simulink library "rtwdemo_pi_controller"  (Simulink 7.6)
settings: Solver=ode45  SolverMode=SingleTasking  StartTime=0.0  StopTime=10.0  RelTol=1e-3
undefined symbols (not defined in the file or in its folder): DiscIntNeverNeededParam, I_Gain, I_InErrMap, I_OutMap, P_Gain, P_InErrMap, P_OutMap
settings Model: Creator=The MathWorks Inc.  ExtModeAutoUpdateStatusClock=off

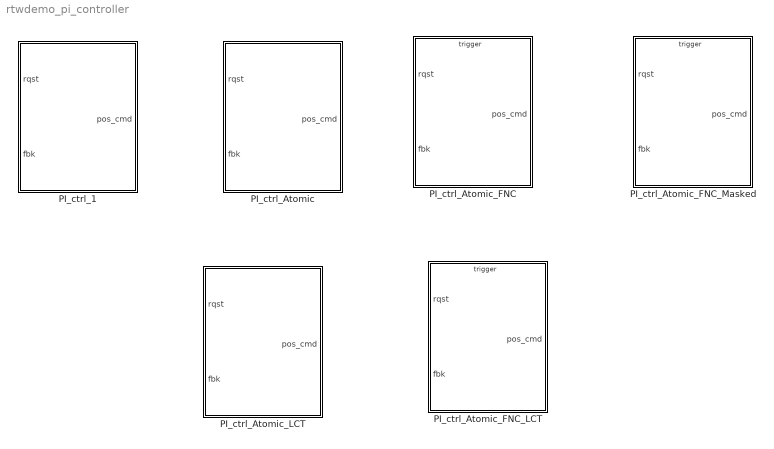
== system rtwdemo_pi_controller ==
  PI_ctrl_1 : Subsystem
      settings: RTWFileNameOpts=Use function name
  PI_ctrl_Atomic : Subsystem  TreatAsAtomicUnit=on  RTWFcnName=PI_Cntrl_Reusable
      settings: RTWFcnNameOpts=User specified  RTWFileNameOpts=Use function name
  PI_ctrl_Atomic_FNC : Subsystem  TreatAsAtomicUnit=on  RTWFcnName=PI_Cntrl_Reusable
      settings: RTWFcnNameOpts=User specified  RTWFileNameOpts=Use function name
  PI_ctrl_Atomic_FNC_LCT : Subsystem  TreatAsAtomicUnit=on  RTWFcnName=PI_Cntrl_Reusable
      settings: RTWFcnNameOpts=User specified  RTWFileNameOpts=Use function name
  PI_ctrl_Atomic_FNC_Masked : Subsystem  TreatAsAtomicUnit=on  RTWFcnName=PI_Cntrl_Reusable  mask{Masked_P_Gain=0, Masked_I_Gain=0}
      mask prompts: Masked_P_Gain "P_Gain"; Masked_I_Gain "I_Gain"
      settings: RTWFcnNameOpts=User specified  RTWFileNameOpts=Use function name
  PI_ctrl_Atomic_LCT : Subsystem  TreatAsAtomicUnit=on  RTWFcnName=PI_Cntrl_Reusable
      settings: RTWFcnNameOpts=User specified  RTWFileNameOpts=Use function name

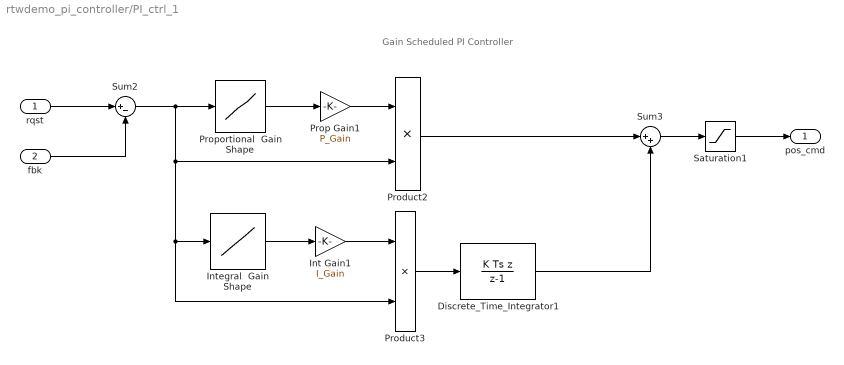
== system rtwdemo_pi_controller/PI_ctrl_1 ==
  note: Gain Scheduled PI Controller
  rqst : Inport
  fbk : Inport  Port=2
  Discrete_Time_Integrator1 : DiscreteIntegrator  IntegratorMethod=Integration: Backward Euler  InitialConditionMode=State only (most efficient)  SampleTime=-1  OutDataTypeStr=Inherit: Inherit via back propagation  UpperSaturationLimit=1  LowerSaturationLimit=-1  ICPrevOutput=DiscIntNeverNeededParam  ICPrevScaledInput=DiscIntNeverNeededParam
  Int Gain1 : Gain  Gain=I_Gain  OutDataTypeStr=Inherit: Same as input  ParamDataTypeStr=Inherit: Same as input
      settings: AttributesFormatString=%<Gain>
  Integral  Gain Shape : Lookup  InputValues=I_InErrMap  Table=I_OutMap
  Product2 : Product  RndMeth=Zero
  Product3 : Product  RndMeth=Zero
  Prop Gain1 : Gain  Gain=P_Gain  OutDataTypeStr=Inherit: Same as input  ParamDataTypeStr=Inherit: Same as input
      settings: AttributesFormatString=%<Gain>
  Proportional  Gain Shape : Lookup  InputValues=P_InErrMap  Table=P_OutMap
  Saturation1 : Saturate  UpperLimit=1  LowerLimit=-1
  Sum2 : Sum  Inputs=|+-  InputSameDT=on
  Sum3 : Sum  Inputs=|++  InputSameDT=on
  pos_cmd : Outport
  wires:
  Discrete_Time_Integrator1/1 -> Sum3/2
  Sum3/1 -> Saturation1/1
  Saturation1/1 -> pos_cmd/1
  rqst/1 -> Sum2/1
  fbk/1 -> Sum2/2
  Sum2/1 -> Product2/2, Product3/2, Integral  Gain Shape/1, Proportional  Gain Shape/1
  Integral  Gain Shape/1 -> Int Gain1/1
  Proportional  Gain Shape/1 -> Prop Gain1/1
  Int Gain1/1 -> Product3/1
  Product3/1 -> Discrete_Time_Integrator1/1
  Prop Gain1/1 -> Product2/1
  Product2/1 -> Sum3/1

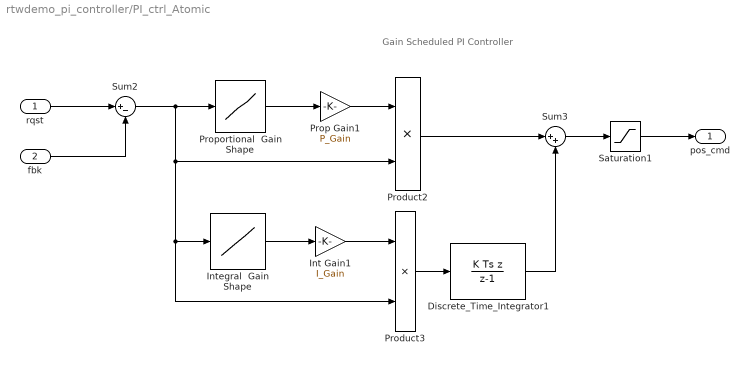
== system rtwdemo_pi_controller/PI_ctrl_Atomic ==
  note: Gain Scheduled PI Controller
  rqst : Inport
  fbk : Inport  Port=2
  Discrete_Time_Integrator1 : DiscreteIntegrator  IntegratorMethod=Integration: Backward Euler  InitialConditionMode=State only (most efficient)  SampleTime=-1  OutDataTypeStr=Inherit: Inherit via back propagation  UpperSaturationLimit=1  LowerSaturationLimit=-1  ICPrevOutput=DiscIntNeverNeededParam  ICPrevScaledInput=DiscIntNeverNeededParam
  Int Gain1 : Gain  Gain=I_Gain  OutDataTypeStr=Inherit: Same as input  ParamDataTypeStr=Inherit: Same as input
      settings: AttributesFormatString=%<Gain>
  Integral  Gain Shape : Lookup  InputValues=I_InErrMap  Table=I_OutMap
  Product2 : Product  RndMeth=Zero
  Product3 : Product  RndMeth=Zero
  Prop Gain1 : Gain  Gain=P_Gain  OutDataTypeStr=Inherit: Same as input  ParamDataTypeStr=Inherit: Same as input
      settings: AttributesFormatString=%<Gain>
  Proportional  Gain Shape : Lookup  InputValues=P_InErrMap  Table=P_OutMap
  Saturation1 : Saturate  UpperLimit=1  LowerLimit=-1
  Sum2 : Sum  Inputs=|+-  InputSameDT=on
  Sum3 : Sum  Inputs=|++  InputSameDT=on
  pos_cmd : Outport
  wires:
  Product2/1 -> Sum3/1
  Prop Gain1/1 -> Product2/1
  Product3/1 -> Discrete_Time_Integrator1/1
  Int Gain1/1 -> Product3/1
  Proportional  Gain Shape/1 -> Prop Gain1/1
  Integral  Gain Shape/1 -> Int Gain1/1
  Sum2/1 -> Proportional  Gain Shape/1, Integral  Gain Shape/1, Product3/2, Product2/2
  fbk/1 -> Sum2/2
  rqst/1 -> Sum2/1
  Saturation1/1 -> pos_cmd/1
  Sum3/1 -> Saturation1/1
  Discrete_Time_Integrator1/1 -> Sum3/2

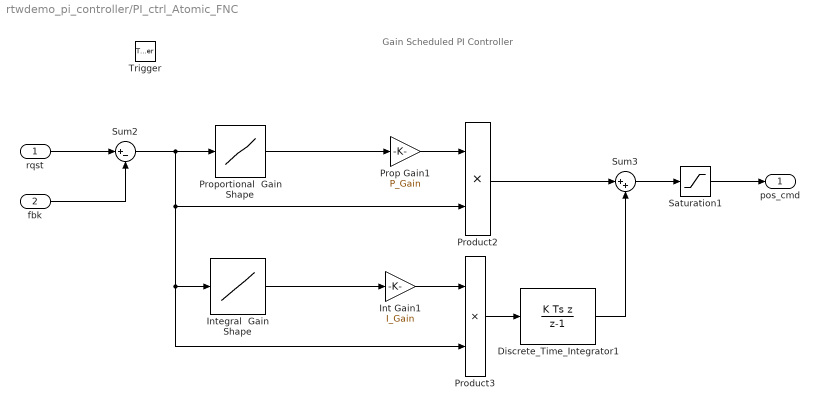
== system rtwdemo_pi_controller/PI_ctrl_Atomic_FNC ==
  note: Gain Scheduled PI Controller
  rqst : Inport
  fbk : Inport  Port=2
  Trigger : TriggerPort  TriggerType=function-call  SampleTimeType=periodic  SampleTime=.001
  Discrete_Time_Integrator1 : DiscreteIntegrator  IntegratorMethod=Integration: Backward Euler  InitialConditionMode=State only (most efficient)  SampleTime=-1  OutDataTypeStr=Inherit: Inherit via back propagation  UpperSaturationLimit=1  LowerSaturationLimit=-1  ICPrevOutput=DiscIntNeverNeededParam  ICPrevScaledInput=DiscIntNeverNeededParam
  Int Gain1 : Gain  Gain=I_Gain  OutDataTypeStr=Inherit: Same as input  ParamDataTypeStr=Inherit: Same as input
      settings: AttributesFormatString=%<Gain>
  Integral  Gain Shape : Lookup  InputValues=I_InErrMap  Table=I_OutMap
  Product2 : Product  RndMeth=Zero
  Product3 : Product  RndMeth=Zero
  Prop Gain1 : Gain  Gain=P_Gain  OutDataTypeStr=Inherit: Same as input  ParamDataTypeStr=Inherit: Same as input
      settings: AttributesFormatString=%<Gain>
  Proportional  Gain Shape : Lookup  InputValues=P_InErrMap  Table=P_OutMap
  Saturation1 : Saturate  UpperLimit=1  LowerLimit=-1
  Sum2 : Sum  Inputs=|+-  InputSameDT=on
  Sum3 : Sum  Inputs=|++  InputSameDT=on
  pos_cmd : Outport
  wires:
  Discrete_Time_Integrator1/1 -> Sum3/2
  Sum3/1 -> Saturation1/1
  Saturation1/1 -> pos_cmd/1
  rqst/1 -> Sum2/1
  fbk/1 -> Sum2/2
  Sum2/1 -> Product2/2, Product3/2, Integral  Gain Shape/1, Proportional  Gain Shape/1
  Integral  Gain Shape/1 -> Int Gain1/1
  Proportional  Gain Shape/1 -> Prop Gain1/1
  Int Gain1/1 -> Product3/1
  Product3/1 -> Discrete_Time_Integrator1/1
  Prop Gain1/1 -> Product2/1
  Product2/1 -> Sum3/1

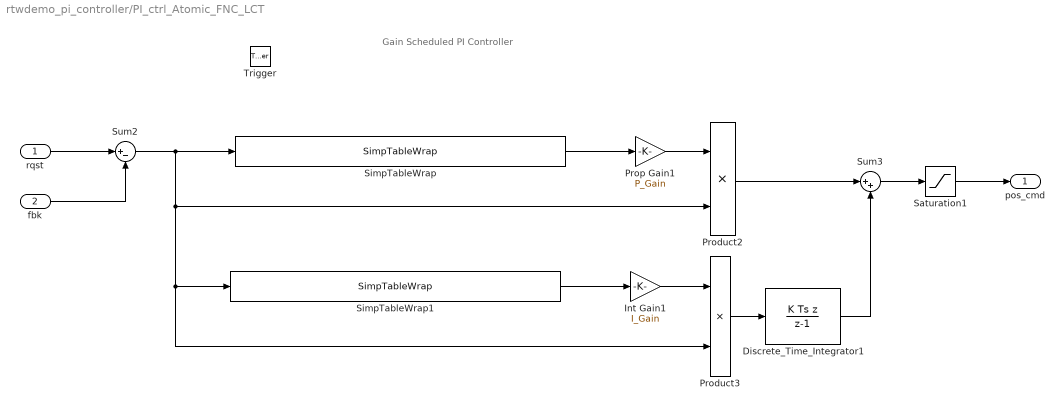
== system rtwdemo_pi_controller/PI_ctrl_Atomic_FNC_LCT ==
  note: Gain Scheduled PI Controller
  rqst : Inport
  fbk : Inport  Port=2
  Trigger : TriggerPort  TriggerType=function-call  SampleTimeType=periodic  SampleTime=.001
  Discrete_Time_Integrator1 : DiscreteIntegrator  IntegratorMethod=Integration: Backward Euler  InitialConditionMode=State only (most efficient)  SampleTime=-1  OutDataTypeStr=Inherit: Inherit via back propagation  UpperSaturationLimit=1  LowerSaturationLimit=-1  ICPrevOutput=DiscIntNeverNeededParam  ICPrevScaledInput=DiscIntNeverNeededParam
  Int Gain1 : Gain  Gain=I_Gain  OutDataTypeStr=Inherit: Same as input  ParamDataTypeStr=Inherit: Same as input
      settings: AttributesFormatString=%<Gain>
  Product2 : Product  RndMeth=Zero
  Product3 : Product  RndMeth=Zero
  Prop Gain1 : Gain  Gain=P_Gain  OutDataTypeStr=Inherit: Same as input  ParamDataTypeStr=Inherit: Same as input
      settings: AttributesFormatString=%<Gain>
  Saturation1 : Saturate  UpperLimit=1  LowerLimit=-1
  SimpTableWrap : S-Function  FunctionName=SimpTableWrap  Parameters=SParameter1, SParameter2, SParameter3  EnableBusSupport=off  mask(Legacy Function){SFunctionSpec=double y1 = SimpleTable(double u1, double p1[], double p2[], int16 p3), SParameter1=P_InErrMap, SParameter2=P_OutMap, SParameter3=int16(length(P_OutMap)), ShowSpec=on}
      mask prompts: SParameter1 "P1:"; SParameter2 "P2:"; SParameter3 "P3:"; ShowSpec "Display function specification"
      mask help:
      | This block allows the user to call the following C function(s) in Simulink:
      |
      | StartFcn: none
      |
      | OutputFcn: double y1 = SimpleTable(double u1, double p1[], double p2[], int16 p3)
      |
      | TerminateFcn: none
      mask CallbackString:
      | ||||if strcmp(get_param(gcbh, 'ShowSpec'), 'on')
      |   set_param(gcbh, 'MaskDisplay', sprintf('fprintf(''%s'');', get_param(gcbh, 'SFunctionSpec')));
      | else
      |   set_param(gcbh, 'MaskDisplay', sprintf('fprintf(''%s'');', get_param(gcbh, 'FunctionName')));
      | end
      mask Display: fprintf('double y1 = SimpleTable(double u1, double p1[], double p2[], int16 p3)');
  SimpTableWrap1 : S-Function  FunctionName=SimpTableWrap  Parameters=SParameter1, SParameter2, SParameter3  EnableBusSupport=off  mask(Legacy Function){SFunctionSpec=double y1 = SimpleTable(double u1, double p1[], double p2[], int16 p3), SParameter1=I_InErrMap, SParameter2=I_OutMap, SParameter3=int16(length(I_OutMap)), ShowSpec=on}
      mask prompts: SParameter1 "P1:"; SParameter2 "P2:"; SParameter3 "P3:"; ShowSpec "Display function specification"
      mask help:
      | This block allows the user to call the following C function(s) in Simulink:
      |
      | StartFcn: none
      |
      | OutputFcn: double y1 = SimpleTable(double u1, double p1[], double p2[], int16 p3)
      |
      | TerminateFcn: none
      mask CallbackString:
      | ||||if strcmp(get_param(gcbh, 'ShowSpec'), 'on')
      |   set_param(gcbh, 'MaskDisplay', sprintf('fprintf(''%s'');', get_param(gcbh, 'SFunctionSpec')));
      | else
      |   set_param(gcbh, 'MaskDisplay', sprintf('fprintf(''%s'');', get_param(gcbh, 'FunctionName')));
      | end
      mask Display: fprintf('double y1 = SimpleTable(double u1, double p1[], double p2[], int16 p3)');
  Sum2 : Sum  Inputs=|+-  InputSameDT=on
  Sum3 : Sum  Inputs=|++  InputSameDT=on
  pos_cmd : Outport
  wires:
  Product2/1 -> Sum3/1
  Prop Gain1/1 -> Product2/1
  Product3/1 -> Discrete_Time_Integrator1/1
  Int Gain1/1 -> Product3/1
  SimpTableWrap/1 -> Prop Gain1/1
  Sum2/1 -> Product2/2, Product3/2, SimpTableWrap1/1, SimpTableWrap/1
  fbk/1 -> Sum2/2
  rqst/1 -> Sum2/1
  Saturation1/1 -> pos_cmd/1
  Sum3/1 -> Saturation1/1
  Discrete_Time_Integrator1/1 -> Sum3/2
  SimpTableWrap1/1 -> Int Gain1/1

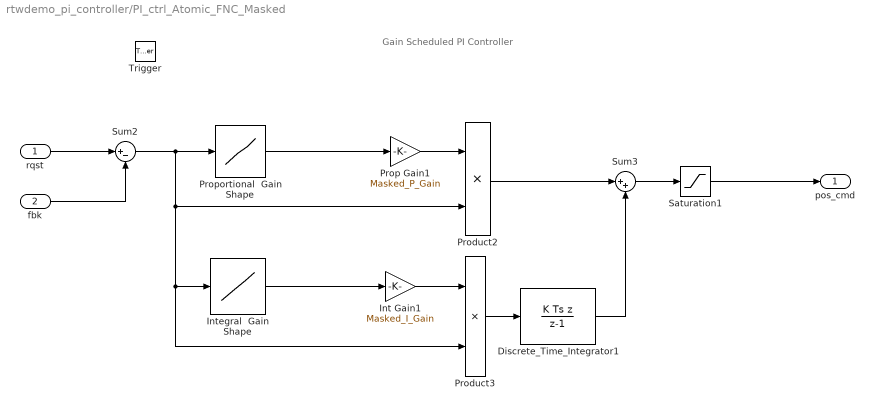
== system rtwdemo_pi_controller/PI_ctrl_Atomic_FNC_Masked ==
  note: Gain Scheduled PI Controller
  rqst : Inport
  fbk : Inport  Port=2
  Trigger : TriggerPort  TriggerType=function-call  SampleTimeType=periodic  SampleTime=.001
  Discrete_Time_Integrator1 : DiscreteIntegrator  IntegratorMethod=Integration: Backward Euler  InitialConditionMode=State only (most efficient)  SampleTime=-1  OutDataTypeStr=Inherit: Inherit via back propagation  UpperSaturationLimit=1  LowerSaturationLimit=-1  ICPrevOutput=DiscIntNeverNeededParam  ICPrevScaledInput=DiscIntNeverNeededParam
  Int Gain1 : Gain  Gain=Masked_I_Gain  OutDataTypeStr=Inherit: Same as input  ParamDataTypeStr=Inherit: Same as input
      settings: AttributesFormatString=%<Gain>
  Integral  Gain Shape : Lookup  InputValues=I_InErrMap  Table=I_OutMap
  Product2 : Product  RndMeth=Zero
  Product3 : Product  RndMeth=Zero
  Prop Gain1 : Gain  Gain=Masked_P_Gain  OutDataTypeStr=Inherit: Same as input  ParamDataTypeStr=Inherit: Same as input
      settings: AttributesFormatString=%<Gain>
  Proportional  Gain Shape : Lookup  InputValues=P_InErrMap  Table=P_OutMap
  Saturation1 : Saturate  UpperLimit=1  LowerLimit=-1
  Sum2 : Sum  Inputs=|+-  InputSameDT=on
  Sum3 : Sum  Inputs=|++  InputSameDT=on
  pos_cmd : Outport
  wires:
  Product2/1 -> Sum3/1
  Prop Gain1/1 -> Product2/1
  Product3/1 -> Discrete_Time_Integrator1/1
  Int Gain1/1 -> Product3/1
  Proportional  Gain Shape/1 -> Prop Gain1/1
  Integral  Gain Shape/1 -> Int Gain1/1
  Sum2/1 -> Proportional  Gain Shape/1, Integral  Gain Shape/1, Product3/2, Product2/2
  fbk/1 -> Sum2/2
  rqst/1 -> Sum2/1
  Saturation1/1 -> pos_cmd/1
  Sum3/1 -> Saturation1/1
  Discrete_Time_Integrator1/1 -> Sum3/2

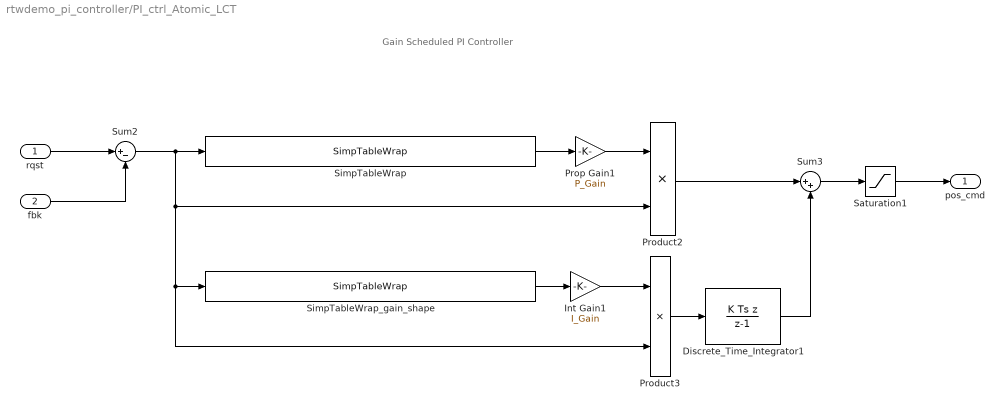
== system rtwdemo_pi_controller/PI_ctrl_Atomic_LCT ==
  note: Gain Scheduled PI Controller
  rqst : Inport
  fbk : Inport  Port=2
  Discrete_Time_Integrator1 : DiscreteIntegrator  IntegratorMethod=Integration: Backward Euler  InitialConditionMode=State only (most efficient)  SampleTime=-1  OutDataTypeStr=Inherit: Inherit via back propagation  UpperSaturationLimit=1  LowerSaturationLimit=-1  ICPrevOutput=DiscIntNeverNeededParam  ICPrevScaledInput=DiscIntNeverNeededParam
  Int Gain1 : Gain  Gain=I_Gain  OutDataTypeStr=Inherit: Same as input  ParamDataTypeStr=Inherit: Same as input
      settings: AttributesFormatString=%<Gain>
  Product2 : Product  RndMeth=Zero
  Product3 : Product  RndMeth=Zero
  Prop Gain1 : Gain  Gain=P_Gain  OutDataTypeStr=Inherit: Same as input  ParamDataTypeStr=Inherit: Same as input
      settings: AttributesFormatString=%<Gain>
  Saturation1 : Saturate  UpperLimit=1  LowerLimit=-1
  SimpTableWrap : S-Function  FunctionName=SimpTableWrap  Parameters=SParameter1, SParameter2, SParameter3  EnableBusSupport=off  mask(Legacy Function){SFunctionSpec=double y1 = SimpleTable(double u1, double p1[], double p2[], int16 p3), SParameter1=P_InErrMap, SParameter2=P_OutMap, SParameter3=int16(length(P_OutMap)), ShowSpec=on}
      mask prompts: SParameter1 "P1:"; SParameter2 "P2:"; SParameter3 "P3:"; ShowSpec "Display function specification"
      mask help:
      | This block allows the user to call the following C function(s) in Simulink:
      |
      | StartFcn: none
      |
      | OutputFcn: double y1 = SimpleTable(double u1, double p1[], double p2[], int16 p3)
      |
      | TerminateFcn: none
      mask CallbackString:
      | ||||if strcmp(get_param(gcbh, 'ShowSpec'), 'on')
      |   set_param(gcbh, 'MaskDisplay', sprintf('fprintf(''%s'');', get_param(gcbh, 'SFunctionSpec')));
      | else
      |   set_param(gcbh, 'MaskDisplay', sprintf('fprintf(''%s'');', get_param(gcbh, 'FunctionName')));
      | end
      mask Display: fprintf('double y1 = SimpleTable(double u1, double p1[], double p2[], int16 p3)');
  SimpTableWrap_gain_shape : S-Function  FunctionName=SimpTableWrap  Parameters=SParameter1, SParameter2, SParameter3  EnableBusSupport=off  mask(Legacy Function){SFunctionSpec=double y1 = SimpleTable(double u1, double p1[], double p2[], int16 p3), SParameter1=I_InErrMap, SParameter2=I_OutMap, SParameter3=int16(length(I_OutMap)), ShowSpec=on}
      mask prompts: SParameter1 "P1:"; SParameter2 "P2:"; SParameter3 "P3:"; ShowSpec "Display function specification"
      mask help:
      | This block allows the user to call the following C function(s) in Simulink:
      |
      | StartFcn: none
      |
      | OutputFcn: double y1 = SimpleTable(double u1, double p1[], double p2[], int16 p3)
      |
      | TerminateFcn: none
      mask CallbackString:
      | ||||if strcmp(get_param(gcbh, 'ShowSpec'), 'on')
      |   set_param(gcbh, 'MaskDisplay', sprintf('fprintf(''%s'');', get_param(gcbh, 'SFunctionSpec')));
      | else
      |   set_param(gcbh, 'MaskDisplay', sprintf('fprintf(''%s'');', get_param(gcbh, 'FunctionName')));
      | end
      mask Display: fprintf('double y1 = SimpleTable(double u1, double p1[], double p2[], int16 p3)');
  Sum2 : Sum  Inputs=|+-  InputSameDT=on
  Sum3 : Sum  Inputs=|++  InputSameDT=on
  pos_cmd : Outport
  wires:
  SimpTableWrap_gain_shape/1 -> Int Gain1/1
  Discrete_Time_Integrator1/1 -> Sum3/2
  Sum3/1 -> Saturation1/1
  Saturation1/1 -> pos_cmd/1
  rqst/1 -> Sum2/1
  fbk/1 -> Sum2/2
  Sum2/1 -> SimpTableWrap/1, SimpTableWrap_gain_shape/1, Product3/2, Product2/2
  SimpTableWrap/1 -> Prop Gain1/1
  Int Gain1/1 -> Product3/1
  Product3/1 -> Discrete_Time_Integrator1/1
  Prop Gain1/1 -> Product2/1
  Product2/1 -> Sum3/1
